simulink model "m01_PMSM_Desktop"  (R2023b)
settings: Solver=FixedStepAuto  StartTime=0.0  StopTime=0.6  FixedStep=Ts  RelTol=1e-3  AbsTol=1e-3
PreLoadFcn:
  | control_data;
  | pmsm_data;
undefined symbols (not defined in the file): avgFactor, Gs, J, Tmax, Ts, Tsc
libraries: fl_lib x54, nesl_utility x53, ee_lib x13, SimscapeFPGAHIL_lib x12, eePmsmFieldOrientedControl x1
(part 1 of 2)
Description:
  | Three-Phase PMSM Drive
settings Model: Creator=The MathWorks, Inc.  LastModifiedBy=promero
settings SolverCC: AutoScaleAbsTol=off  MaxConsecutiveMinStep=2  ZeroCrossAlgorithm=Adaptive  AlgebraicLoopSolver=TrustRegion  MaxZcPerStep=1
settings DataIOCC: MaxDataPoints=690000  SaveOutput=off  DSMLogging=off  SaveTime=off
settings OptimizationCC: ReuseModelBlockBuffer=off  LifeSpan=inf
settings DebuggingCC: UnderspecifiedInitializationDetection=Classic  MergeDetectMultiDrivingBlocksExec=none  MaxConsecutiveZCsMsg=none  IgnoredZcDiagnostic=none  InheritedTsInSrcMsg=none  UnconnectedInputMsg=warning  UnconnectedOutputMsg=warning  UnconnectedLineMsg=warning  AllowSymbolicDim=off  PregeneratedLibrarySubsystemCodeDiagnostic=none  SFUnexpectedBacktrackingDiag=warning  SFNoUnconditionalDefaultTransitionDiag=warning  SFExecutionAtInitializationDiag=none  ArithmeticOperatorsInVariantConditions=warning
settings HardwareCC: ProdBitPerPointer=32  ProdBitPerSizeT=32  ProdBitPerPtrDiffT=32  ProdLargestAtomicFloat=None  ProdIntDivRoundTo=Undefined  ProdEndianess=Unspecified  ProdWordSize=32  ProdHWDeviceType=ASIC/FPGA->ASIC/FPGA  TargetBitPerPointer=64  TargetBitPerSizeT=64  TargetBitPerPtrDiffT=64  TargetLongLongMode=on  TargetIntDivRoundTo=Zero  TargetEndianess=LittleEndian  TargetWordSize=64  TargetHWDeviceType=Custom Processor->MATLAB Host Computer  ProdEqTarget=off
settings ModelReferenceCC: EnableRefExpFcnMdlSchedulingChecks=on  PropagateSignalLabelsOutOfModel=off
settings SFSimCC: SimUseLocalCustomCode=off
settings RTWCC: RTWUseLocalCustomCode=off  DLArmComputeVersion=19.05
settings CodeAppCC: StateflowObjectComments=on
settings GRTTargetCC: TargetLangStandard=C89/C90 (ANSI)
settings ConfigComp: CovMetricSettings=dw  CovSaveCumulativeToWorkspaceVar=on  CovSaveSingleToWorkspaceVar=on  CovExternalEMLEnable=off  CovSFcnEnable=off
settings SimscapeCC: SimscapeLogSimulationStatistics=on  SimscapeLogName=simlog_ee_pmsm_drive  SimscapeLogDataHistory=690000

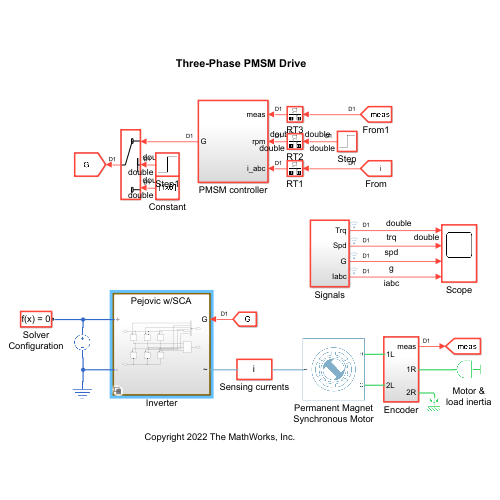
[thumbnail: Simulink's stored preview of the top-level diagram]
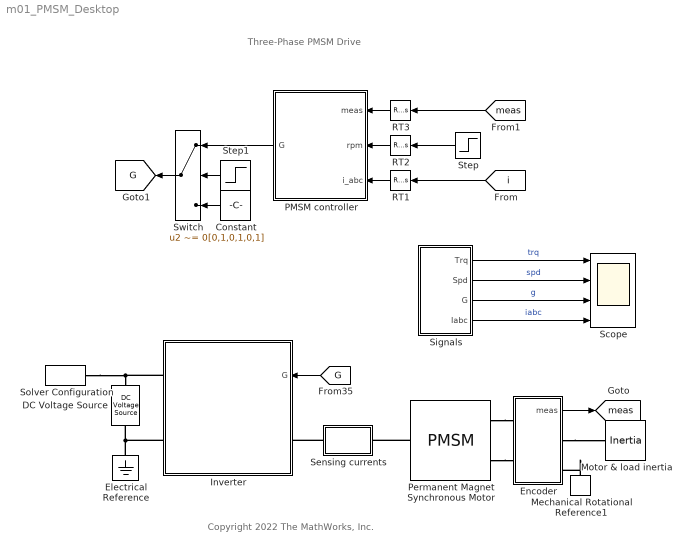
== system m01_PMSM_Desktop ==
  note: Three-Phase PMSM Drive
  note: Copyright 2022 The MathWorks, Inc.
  Constant : Constant  Value=[0,1,0,1,0,1]  SampleTime=-1
  DC Voltage Source : fl_lib/Electrical/Electrical Sources/DC Voltage Source  v0=48 V
  Electrical Reference : fl_lib/Electrical/Electrical Elements/Electrical Reference
  Encoder : Subsystem
  Inverter : Subsystem  Variant=on  VariantControlMode=label  VariantControl=Choice  LabelModeActiveChoice=PejovicSCA
  Mechanical Rotational Reference1 : fl_lib/Mechanical/Rotational Elements/Mechanical Rotational Reference
  Motor & load inertia : fl_lib/Mechanical/Rotational Elements/Inertia  inertia=J kg*m^2  num_ports=foundation.enum.numPorts2.one  w_specify=on  w_priority=High  w=0 rpm  w_nominal_specify=off  w_nominal_unit=rad/s  w_nominal_value=1  t_specify=off  t_priority=High  t=0 N*m  t_nominal_specify=off  t_nominal_unit=N*m  t_nominal_value=1
  PMSM controller : Subsystem
  Permanent Magnet Synchronous Motor : ee_lib/Electromechanical/Permanent Magnet/PMSM  port_option=ee.enum.threePhasePort.composite  winding_type=ee.enum.statorconnection.wye  machine_param=ee.enum.pmsm.parameterization.constant  nPolePairs=N  pmflux_param=ee.enum.pmflux.fluxlinkage  pm_flux_linkage=PM Wb  torque_constant=0.18 N*m/A  back_emf_constant=0.18 V/(rad/s)  stator_param=ee.enum.statorparam.LdLqL0  Ld=Ld H  Lq=Lq H  idVec=[-200, 0, 200] A  iqVec=[-200, 0, 200] A  LdMatrix=0.0002 * ones(3, 3) H  LqMatrix=0.0002 * ones(3, 3) H  PmMatrix=0.1 * ones(3, 3) Wb  ktMatrix=0.18 * ones(3, 3) N*m/A  keMatrix=0.18 * ones(3, 3) V/(rad/s)  L0=L0 H  Ls=0.0002 H  Lm=0.00002 H  Ms=0.00002 H  Rs=Rs Ohm  zero_sequence=ee.enum.park.zerosequence.exclude  axes_param=ee.enum.rotorangle.qaxis  loss_param=ee.enum.ironloss.none  losses_oc=[0, 0, 0] W  losses_sc=[0, 0, 0] W  f_losses=60 Hz  Isc_losses=95 A  J=0 kg*m^2  lam=0 N*m/(rad/s)  i_d_specify=off  i_d_priority=None  i_d=0 A  i_d_nominal_specify=off  i_d_nominal_unit=A  i_d_nominal_value=1  i_q_specify=off  i_q_priority=None  i_q=0 A  i_q_nominal_specify=off  i_q_nominal_unit=A  i_q_nominal_value=1  torque_specify=off  torque_priority=None  torque=0 N*m  torque_nominal_specify=off  torque_nominal_unit=N*m  torque_nominal_value=1  angular_velocity_specify=on  angular_velocity_priority=None  angular_velocity=0 rpm  angular_velocity_nominal_specify=off  angular_velocity_nominal_unit=rpm  angular_velocity_nominal_value=1  angular_position_specify=on  angular_position_priority=High  angular_position=0 rad  angular_position_nominal_specify=off  angular_position_nominal_unit=deg  angular_position_nominal_value=1  alpha=3.93e-3 1/K  alpha_flux=-0.001 1/K  Tmeas=298.15 K  stator_thermal_mass=100 J/K  rotor_thermal_mass=200 J/K  Rm_percent_rotor=90  Rd_percent_rotor=30  temperatureA_specify=off  temperatureA_priority=High  temperatureA=25 degC  temperatureA_nominal_specify=off  temperatureA_nominal_unit=degC  temperatureA_nominal_value=1  temperatureB_specify=off  temperatureB_priority=High  temperatureB=25 degC  temperatureB_nominal_specify=off  temperatureB_nominal_unit=degC  temperatureB_nominal_value=1  temperatureC_specify=off  temperatureC_priority=High  temperatureC=25 degC  temperatureC_nominal_specify=off  temperatureC_nominal_unit=degC  temperatureC_nominal_value=1  temperatureR_specify=off  temperatureR_priority=High  temperatureR=25 degC  temperatureR_nominal_specify=off  temperatureR_nominal_unit=degC  temperatureR_nominal_value=1
      settings: InternalSimscapePortConfiguration="{\"Bottom\":[],\"Left\":[{\"id\":\"N\",\"label\":\"~\",\"type\":\"foundation.electrical.three_phase\"}],\"Right\":[{\"id\":\"R\",\"label\":\"R\",\"type\":\"foundation.mechanical.rotational.rotational\"},{\"id\":\"C\",\"label\":\"C\",\"type\":\"foundation.mechanical.rotational.rotational\"}],\"Top\":[]}"
  RT1 : RateTransition  OutPortSampleTime=Tsc
  RT2 : RateTransition  OutPortSampleTime=Tsc
  RT3 : RateTransition  OutPortSampleTime=Tsc
  Scope : Scope  NumInputPorts=4
  Sensing currents : Subsystem
      mask Display: disp('i')
  "Signals " : Subsystem
  Solver Configuration : nesl_utility/Solver Configuration  PhysicalDomain=network_engine_domain  SubClassName=solver  LeftPortType=input  RightPortType=generic  Tones=[]  Harmonics=[]  SimulateNoise=off  Profile=off  UseLocalSampling=off  EnableSwitchedLinearOptims=on  FrequencyDomain=off  UseCCode=off  RelTol=0.001  AbsTol=1e-06  MinStep=1e-09  ToWorkspace=off  RevertToSquareIcSolve=off  NumHomotopyIterations=100  PhasorMode=off  PhasorModeNumHarmonics=1  ConsistencySolver=NEWTON_FTOL  IndexReductionMethod=DerivativeReplacement  DoDC=off  ResidualTolerance=1e-9  ConsistencyTolSource=GLOBAL  ConsistencyAbsTol=0.001  ConsistencyRelTol=0.001  ConsistencyTolFactor=0.001  UseLocalSolver=on  LocalSolverChoice=NE_PARTITIONING_ADVANCER  ResolveIndetEquations=on  FunctionEvalNumThread=1  LocalSolverSampleTime=Ts  DoFixedCost=off  MaxNonlinIter=1  MaxModeIter=2  ComputeImpulses=off  ImpulseIterations=2  LinearAlgebra=auto  LinearAlgebraNumThread=0  EquationFormulation=NE_TIME_EF  DelaysMemoryBudget=1024  AutomaticFiltering=on  FilteringTimeConstant=0.001  PartitionStorageMethod=AS_NEEDED  PartitionMemoryBudget=1024  PartitionMethod=FAST  MultibodyUseLocalSolver=off  MultibodyLocalSolverChoice=ODE1  MultibodyLocalSolverSampleTime=0.001
  Step : Step  Time=0.1  After=500  SampleTime=Tsc
  Step1 : Step  Time=1e-4
  Switch : Switch  Criteria=u2 ~= 0  SaturateOnIntegerOverflow=off  InputSameDT=off
  tag scope: G=global, meas=global
  wires:
  Step/1 -> RT2/1
  RT3/1 -> PMSM controller/1(meas)
  RT2/1 -> PMSM controller/2(rpm)
  RT1/1 -> PMSM controller/3(i_abc)
  "Signals "/2(Spd) -> Scope/2  "spd"
  "Signals "/4(Iabc) -> Scope/4  "iabc"
  "Signals "/3(G) -> Scope/3  "g"
  "Signals "/1(Trq) -> Scope/1  "trq"
  [i] -> RT1/1
  Encoder/1(meas) -> [meas]
  [meas] -> RT3/1
  PMSM controller/1(G) -> Switch/1
  Constant/1 -> Switch/3
  Step1/1 -> Switch/2
  Switch/1 -> [G]
  [G] -> Inverter/1(G)
  connections:
  Permanent Magnet Synchronous Motor/RConn1 -- Encoder/LConn1
  Permanent Magnet Synchronous Motor/RConn2 -- Encoder/LConn2
  Encoder/RConn1 -- Motor & load inertia/LConn1
  Mechanical Rotational Reference1/LConn1 -- Encoder/RConn2
  Permanent Magnet Synchronous Motor/LConn1 -- Sensing currents/RConn1
  Solver Configuration/RConn1 -- DC Voltage Source/LConn1 -- Inverter/RConn1
  DC Voltage Source/RConn1 -- Inverter/RConn2 -- Electrical Reference/LConn1
  Sensing currents/LConn1 -- Inverter/LConn1

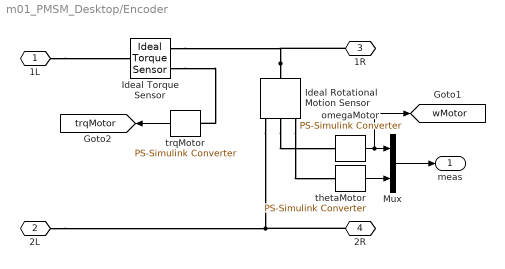
== system m01_PMSM_Desktop/Encoder ==
  Ideal Rotational Motion Sensor : fl_lib/Mechanical/Mechanical Sensors/Ideal Rotational Motion Sensor  reference=foundation.enum.MeasurementReference.difference  acceleration_port=false  velocity_port=true  position_port=true  wrap_angle=simscape.enum.onoff.off  offset=0 deg
  Ideal Torque Sensor : fl_lib/Mechanical/Mechanical Sensors/Ideal Torque Sensor
  Mux : Mux  Inputs=2
  omegaMotor : nesl_utility/PS-Simulink Converter  PhysicalDomain=network_engine_domain  SubClassName=ps_output  LeftPortType=input  RightPortType=output  PseudoPeriodic=off  Frequencies=[]  VectorFormat=1-D array  Unit=inherit  AffineConversion=off
  thetaMotor : nesl_utility/PS-Simulink Converter  PhysicalDomain=network_engine_domain  SubClassName=ps_output  LeftPortType=input  RightPortType=output  PseudoPeriodic=off  Frequencies=[]  VectorFormat=1-D array  Unit=inherit  AffineConversion=off
  trqMotor : nesl_utility/PS-Simulink Converter  PhysicalDomain=network_engine_domain  SubClassName=ps_output  LeftPortType=input  RightPortType=output  PseudoPeriodic=off  Frequencies=[]  VectorFormat=1-D array  Unit=inherit  AffineConversion=off
  1L : PMIOPort  Side=Left
  2L : PMIOPort  Port=2  Side=Left
  1R : PMIOPort  Port=3  Side=Right
  2R : PMIOPort  Port=4  Side=Right
  meas : Outport  VectorParamsAs1DForOutWhenUnconnected=off
  tag scope: trqMotor=global, wMotor=global
  wires:
  trqMotor/1 -> [trqMotor]
  Mux/1 -> meas/1
  thetaMotor/1 -> Mux/2
  omegaMotor/1 -> [wMotor], Mux/1
  connections:
  Ideal Torque Sensor/RConn2 -- trqMotor/LConn1
  1L/RConn1 -- Ideal Torque Sensor/LConn1
  2R/RConn1 -- 2L/RConn1 -- Ideal Rotational Motion Sensor/RConn1
  Ideal Rotational Motion Sensor/LConn1 -- 1R/RConn1 -- Ideal Torque Sensor/RConn1
  Ideal Rotational Motion Sensor/RConn2 -- omegaMotor/LConn1
  Ideal Rotational Motion Sensor/RConn3 -- thetaMotor/LConn1

== system m01_PMSM_Desktop/Inverter ==
  G : Inport
  Pejovic : Subsystem  VariantControl=Pejovic
  Pejovic w/SCA : Subsystem  VariantControl=PejovicSCA
  Simscape Converter : Subsystem  VariantControl=SimscapeConv
  Simscape Switches : Subsystem  VariantControl=SimscapeSw
  + : PMIOPort  Side=Right
  - : PMIOPort  Port=2  Side=Right
  ~ : PMIOPort  Port=3  Side=Left

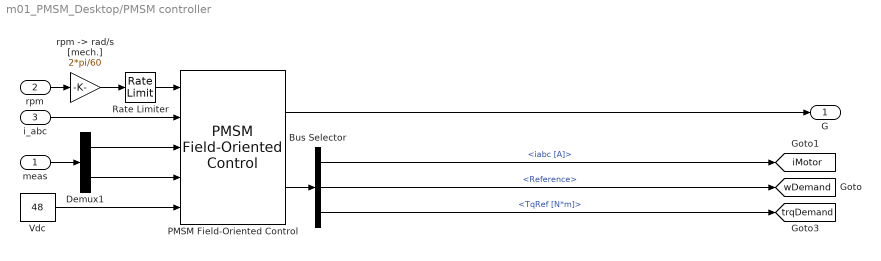
== system m01_PMSM_Desktop/PMSM controller ==
  meas : Inport
  rpm : Inport  Port=2
  i_abc : Inport  Port=3
  Bus Selector : BusSelector  OutputSignals=iabc [A],Reference,TqRef [N*m]
  Demux1 : Demux  Outputs=2
  PMSM Field-Oriented Control : eePmsmFieldOrientedControl/PMSM Field-Oriented Control  winding_type=Wye-wound  CtrlMode=Velocity control  Vnom=48  Pmax=Pmax  Tmax=Tmax*1.5  p=N  Vdc_on=10  Ts=Ts  Tsc=Tsc  CtrlType=PI control  Kp_w=60  Ki_w=300*2  Kv_w=1  Kaw_w=1000  RefType=Zero d-axis control  rpmVec=[0, 3000]  TqVec=[-100, 0, 100]  VdcVec=[300, 350]  PWMMode=SPWM: sinusoidal PWM  ModFactor=1  idMatrix=zeros(2,3,2)  iqMatrix=zeros(2,3,2)  psim=PM  Ld=0.00024  Lq=0.00029  Rs=0.01  AxisAlignment=Q-axis  Kp_id=0.1  Ki_id=10  Kaw_id=1000  Kp_iq=0.1  Ki_iq=10  Kaw_iq=1000  AxisPrio=Q-axis  ActZC=off  ActFF=on  ParamTypeFF=Constant parameters  LdFF=Ld  LqFF=Lq  psimFF=PM  idVect=[-200, 0, 200]  iqVect=[-200, 0, 200]  LdMatrix=0.0002 * ones(3, 3)  LqMatrix=0.0002 * ones(3, 3)  psimMatrix=0.04 * ones(3, 3)  CPWMMode=SPWM: sinusoidal PWM  fsw=fsw
  Rate Limiter : RateLimiter  RisingSlewLimit=Tmax/J  FallingSlewLimit=-Tmax/J  SampleTimeMode=inherited
  Vdc : Constant  Value=48  SampleTime=Tsc
  "rpm -> rad/s [mech.]" : Gain  Gain=2*pi/60
  G : Outport  VectorParamsAs1DForOutWhenUnconnected=off
  tag scope: iMotor=global, trqDemand=global, wDemand=global
  wires:
  Vdc/1 -> PMSM Field-Oriented Control/5
  PMSM Field-Oriented Control/2 -> Bus Selector/1
  i_abc/1 -> PMSM Field-Oriented Control/2
  meas/1 -> Demux1/1
  Demux1/1 -> PMSM Field-Oriented Control/3
  Demux1/2 -> PMSM Field-Oriented Control/4
  Bus Selector/1 -> [iMotor]  "<iabc [A]>"
  Bus Selector/2 -> [wDemand]  "<Reference>"
  Bus Selector/3 -> [trqDemand]  "<TqRef [N*m]>"
  rpm/1 -> "rpm -> rad/s [mech.]"/1
  Rate Limiter/1 -> PMSM Field-Oriented Control/1
  "rpm -> rad/s [mech.]"/1 -> Rate Limiter/1
  PMSM Field-Oriented Control/1 -> G/1

== system m01_PMSM_Desktop/Sensing currents ==
  Current Sensor : ee_lib/Sensors & Transducers/Current Sensor (Three-Phase)
  Gain : Gain  Commented=through  Gain=1/sqrt(3)
  Iabc : nesl_utility/PS-Simulink Converter  PhysicalDomain=network_engine_domain  SubClassName=ps_output  LeftPortType=input  RightPortType=output  PseudoPeriodic=off  Frequencies=[]  VectorFormat=1-D array  Unit=A  AffineConversion=off
  Conn1 : PMIOPort  Side=Left
  Conn2 : PMIOPort  Port=2  Side=Right
  tag scope: i=global
  wires:
  Iabc/1 -> Gain/1
  Gain/1 -> [i]
  connections:
  Current Sensor/RConn1 -- Iabc/LConn1
  Conn2/RConn1 -- Current Sensor/RConn2
  Current Sensor/LConn1 -- Conn1/RConn1

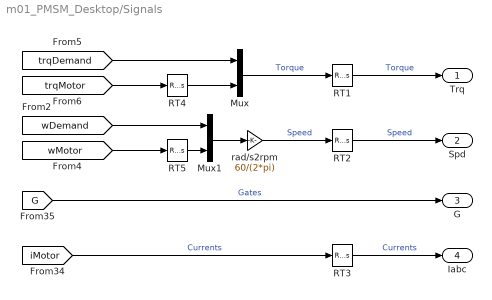
== system m01_PMSM_Desktop/Signals  ==
  Mux : Mux  Inputs=2
  Mux1 : Mux  Inputs=2
  RT1 : RateTransition  OutPortSampleTime=Ts
  RT2 : RateTransition  OutPortSampleTime=Ts
  RT3 : RateTransition  OutPortSampleTime=Ts
  RT4 : RateTransition  OutPortSampleTime=Tsc
  RT5 : RateTransition  OutPortSampleTime=Tsc
  rad/s2rpm : Gain  Gain=60/(2*pi)
  Trq : Outport  VectorParamsAs1DForOutWhenUnconnected=off
  Spd : Outport  Port=2  VectorParamsAs1DForOutWhenUnconnected=off
  G : Outport  Port=3  VectorParamsAs1DForOutWhenUnconnected=off
  Iabc : Outport  Port=4  VectorParamsAs1DForOutWhenUnconnected=off
  wires:
  [trqDemand] -> Mux/1
  [G] -> G/1  "Gates"
  Mux1/1 -> rad/s2rpm/1
  Mux/1 -> RT1/1  "Torque"
  [iMotor] -> RT3/1  "Currents"
  [wDemand] -> Mux1/1
  rad/s2rpm/1 -> RT2/1  "Speed"
  [trqMotor] -> RT4/1
  [wMotor] -> RT5/1
  RT1/1 -> Trq/1  "Torque"
  RT2/1 -> Spd/1  "Speed"
  RT3/1 -> Iabc/1  "Currents"
  RT4/1 -> Mux/2
  RT5/1 -> Mux1/2

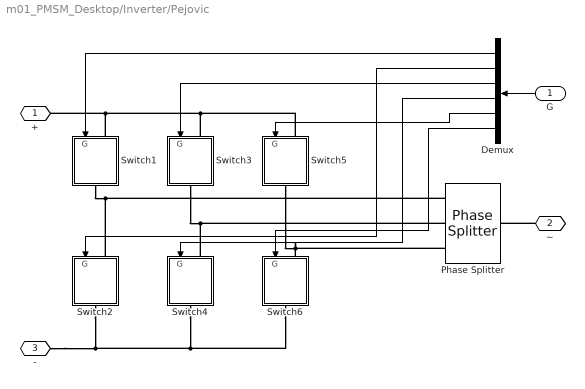
== system m01_PMSM_Desktop/Inverter/Pejovic ==
  G : Inport
  Demux : Demux  Outputs=6
  Phase Splitter : ee_lib/Connectors & References/Phase Splitter
  Switch1 : Subsystem  mask{threshold=0.5, Gs=Gs, timeScaling=1, avgFactor=1}
      mask prompts: threshold "Threshold voltage [V]"; Gs "Conductance (1/Ohm)"; timeScaling "Time scaling"; avgFactor "Subcycle average factor"
      settings: CopyFcn=set_param(gcb, 'LinkStatus', 'none');
  Switch2 : Subsystem  mask{threshold=0.5, Gs=Gs, timeScaling=1, avgFactor=1}
      mask prompts: threshold "Threshold voltage [V]"; Gs "Conductance (1/Ohm)"; timeScaling "Time scaling"; avgFactor "Subcycle average factor"
      settings: CopyFcn=set_param(gcb, 'LinkStatus', 'none');
  Switch3 : Subsystem  mask{threshold=0.5, Gs=Gs, timeScaling=1, avgFactor=1}
      mask prompts: threshold "Threshold voltage [V]"; Gs "Conductance (1/Ohm)"; timeScaling "Time scaling"; avgFactor "Subcycle average factor"
      settings: CopyFcn=set_param(gcb, 'LinkStatus', 'none');
  Switch4 : Subsystem  mask{threshold=0.5, Gs=Gs, timeScaling=1, avgFactor=1}
      mask prompts: threshold "Threshold voltage [V]"; Gs "Conductance (1/Ohm)"; timeScaling "Time scaling"; avgFactor "Subcycle average factor"
      settings: CopyFcn=set_param(gcb, 'LinkStatus', 'none');
  Switch5 : Subsystem  mask{threshold=0.5, Gs=Gs, timeScaling=1, avgFactor=1}
      mask prompts: threshold "Threshold voltage [V]"; Gs "Conductance (1/Ohm)"; timeScaling "Time scaling"; avgFactor "Subcycle average factor"
      settings: CopyFcn=set_param(gcb, 'LinkStatus', 'none');
  Switch6 : Subsystem  mask{threshold=0.5, Gs=Gs, timeScaling=1, avgFactor=1}
      mask prompts: threshold "Threshold voltage [V]"; Gs "Conductance (1/Ohm)"; timeScaling "Time scaling"; avgFactor "Subcycle average factor"
      settings: CopyFcn=set_param(gcb, 'LinkStatus', 'none');
  + : PMIOPort  Side=Right
  ~ : PMIOPort  Port=2  Side=Left
  - : PMIOPort  Port=3  Side=Right
  wires:
  Demux/6 -> Switch6/1(G)
  Demux/5 -> Switch5/1(G)
  Demux/4 -> Switch4/1(G)
  Demux/3 -> Switch3/1(G)
  Demux/2 -> Switch2/1(G)
  Demux/1 -> Switch1/1(G)
  G/1 -> Demux/1
  connections:
  +/RConn1 -- Switch1/LConn1 -- Switch5/LConn1 -- Switch3/LConn1
  Phase Splitter/RConn1 -- Switch2/LConn1 -- Switch1/RConn1
  Switch6/RConn1 -- Switch4/RConn1 -- Switch2/RConn1 -- -/RConn1
  ~/RConn1 -- Phase Splitter/LConn1
  Phase Splitter/RConn2 -- Switch4/LConn1 -- Switch3/RConn1
  Phase Splitter/RConn3 -- Switch6/LConn1 -- Switch5/RConn1

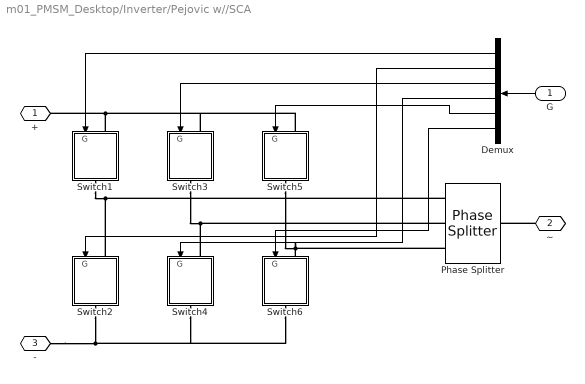
== system m01_PMSM_Desktop/Inverter/Pejovic w//SCA ==
  G : Inport
  Demux : Demux  Outputs=6
  Phase Splitter : ee_lib/Connectors & References/Phase Splitter
  Switch1 : Subsystem  mask{threshold=0.5, Gs=Gs, timeScaling=1, avgFactor=avgFactor}
      mask prompts: threshold "Threshold voltage [V]"; Gs "Conductance (1/Ohm)"; timeScaling "Time scaling"; avgFactor "Subcycle average factor"
      settings: CopyFcn=set_param(gcb, 'LinkStatus', 'none');
  Switch2 : Subsystem  mask{threshold=0.5, Gs=Gs, timeScaling=1, avgFactor=avgFactor}
      mask prompts: threshold "Threshold voltage [V]"; Gs "Conductance (1/Ohm)"; timeScaling "Time scaling"; avgFactor "Subcycle average factor"
      settings: CopyFcn=set_param(gcb, 'LinkStatus', 'none');
  Switch3 : Subsystem  mask{threshold=0.5, Gs=Gs, timeScaling=1, avgFactor=avgFactor}
      mask prompts: threshold "Threshold voltage [V]"; Gs "Conductance (1/Ohm)"; timeScaling "Time scaling"; avgFactor "Subcycle average factor"
      settings: CopyFcn=set_param(gcb, 'LinkStatus', 'none');
  Switch4 : Subsystem  mask{threshold=0.5, Gs=Gs, timeScaling=1, avgFactor=avgFactor}
      mask prompts: threshold "Threshold voltage [V]"; Gs "Conductance (1/Ohm)"; timeScaling "Time scaling"; avgFactor "Subcycle average factor"
      settings: CopyFcn=set_param(gcb, 'LinkStatus', 'none');
  Switch5 : Subsystem  mask{threshold=0.5, Gs=Gs, timeScaling=1, avgFactor=avgFactor}
      mask prompts: threshold "Threshold voltage [V]"; Gs "Conductance (1/Ohm)"; timeScaling "Time scaling"; avgFactor "Subcycle average factor"
      settings: CopyFcn=set_param(gcb, 'LinkStatus', 'none');
  Switch6 : Subsystem  mask{threshold=0.5, Gs=Gs, timeScaling=1, avgFactor=avgFactor}
      mask prompts: threshold "Threshold voltage [V]"; Gs "Conductance (1/Ohm)"; timeScaling "Time scaling"; avgFactor "Subcycle average factor"
      settings: CopyFcn=set_param(gcb, 'LinkStatus', 'none');
  + : PMIOPort  Side=Right
  ~ : PMIOPort  Port=2  Side=Left
  - : PMIOPort  Port=3  Side=Right
  wires:
  G/1 -> Demux/1
  Demux/1 -> Switch1/1(G)
  Demux/2 -> Switch2/1(G)
  Demux/3 -> Switch3/1(G)
  Demux/4 -> Switch4/1(G)
  Demux/5 -> Switch5/1(G)
  Demux/6 -> Switch6/1(G)
  connections:
  Phase Splitter/RConn3 -- Switch6/LConn1 -- Switch5/RConn1
  Phase Splitter/RConn2 -- Switch4/LConn1 -- Switch3/RConn1
  ~/RConn1 -- Phase Splitter/LConn1
  Switch6/RConn1 -- Switch4/RConn1 -- Switch2/RConn1 -- -/RConn1
  Phase Splitter/RConn1 -- Switch2/LConn1 -- Switch1/RConn1
  Switch5/LConn1 -- Switch3/LConn1 -- Switch1/LConn1 -- +/RConn1

== system m01_PMSM_Desktop/Inverter/Simscape Converter ==
  G : Inport
  Converter (Three-Phase) : ee_lib/Semiconductors & Converters/Converters/Converter (Three-Phase)  port_option=ee.enum.threePhasePort.composite  device_type=ee.enum.converters.switchingdevice.ideal  K=0  Vf=0.8 V  Ron=0.001 Ohm  Rds=0.001 Ohm  Goff=1e-6 1/Ohm  Vgt=1 V  Vgt_off=-1 V  Ih=1 A  Vth=0.5 V  diode_param=ee.enum.converters.protectiondiode.none  diode_Vf=0.8 V  diode_Ron=0.001 Ohm  diode_Goff=1e-5 1/Ohm  diode_C=50 nF  diode_iRM=-235 A  diode_iF=300 A  diode_idot=-50 A/us  diode_trr_param=ee.enum.converters.diodetrr.trr_factor  diode_trr_factor=3  diode_trr=15 us  diode_Qrr=1500 s*uA  snubber_type=ee.enum.converters.snubber.exclude  Cs=1e-7 F  Rs=0.1 Ohm
  Gates : Subsystem
  + : PMIOPort  Side=Right
  ~ : PMIOPort  Port=2  Side=Left
  - : PMIOPort  Port=3  Side=Right
  wires:
  G/1 -> Gates/1(Gates Simulink)
  connections:
  -/RConn1 -- Converter (Three-Phase)/RConn2
  Converter (Three-Phase)/RConn1 -- +/RConn1
  Gates/RConn1 -- Converter (Three-Phase)/LConn1
  Converter (Three-Phase)/LConn2 -- ~/RConn1

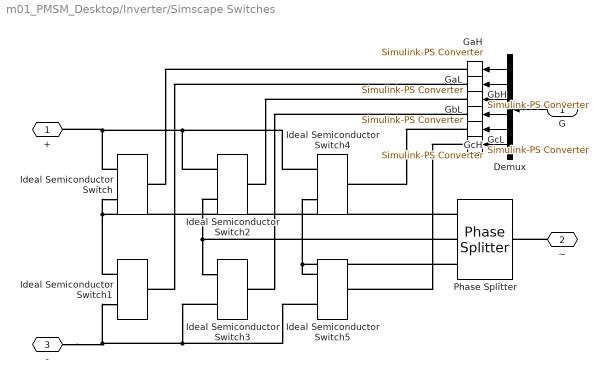
== system m01_PMSM_Desktop/Inverter/Simscape Switches ==
  G : Inport
  Demux : Demux  Outputs=6
  GaH : nesl_utility/Simulink-PS Converter  PhysicalDomain=network_engine_domain  SubClassName=ps_input  LeftPortType=input  RightPortType=output  PseudoPeriodic=off  Frequencies=[]  NoiseDistribution=none  NoiseParameters=[]  Unit=1  AffineConversion=off  FilteringAndDerivatives=zero  SimscapeFilterOrder=1  InputFilterTimeConstant=0.001  UdotUserProvided=0
  GaL : nesl_utility/Simulink-PS Converter  PhysicalDomain=network_engine_domain  SubClassName=ps_input  LeftPortType=input  RightPortType=output  PseudoPeriodic=off  Frequencies=[]  NoiseDistribution=none  NoiseParameters=[]  Unit=1  AffineConversion=off  FilteringAndDerivatives=zero  SimscapeFilterOrder=1  InputFilterTimeConstant=0.001  UdotUserProvided=0
  GbH : nesl_utility/Simulink-PS Converter  PhysicalDomain=network_engine_domain  SubClassName=ps_input  LeftPortType=input  RightPortType=output  PseudoPeriodic=off  Frequencies=[]  NoiseDistribution=none  NoiseParameters=[]  Unit=1  AffineConversion=off  FilteringAndDerivatives=zero  SimscapeFilterOrder=1  InputFilterTimeConstant=0.001  UdotUserProvided=0
  GbL : nesl_utility/Simulink-PS Converter  PhysicalDomain=network_engine_domain  SubClassName=ps_input  LeftPortType=input  RightPortType=output  PseudoPeriodic=off  Frequencies=[]  NoiseDistribution=none  NoiseParameters=[]  Unit=1  AffineConversion=off  FilteringAndDerivatives=zero  SimscapeFilterOrder=1  InputFilterTimeConstant=0.001  UdotUserProvided=0
  GcH : nesl_utility/Simulink-PS Converter  PhysicalDomain=network_engine_domain  SubClassName=ps_input  LeftPortType=input  RightPortType=output  PseudoPeriodic=off  Frequencies=[]  NoiseDistribution=none  NoiseParameters=[]  Unit=1  AffineConversion=off  FilteringAndDerivatives=zero  SimscapeFilterOrder=1  InputFilterTimeConstant=0.001  UdotUserProvided=0
  GcL : nesl_utility/Simulink-PS Converter  PhysicalDomain=network_engine_domain  SubClassName=ps_input  LeftPortType=input  RightPortType=output  PseudoPeriodic=off  Frequencies=[]  NoiseDistribution=none  NoiseParameters=[]  Unit=1  AffineConversion=off  FilteringAndDerivatives=zero  SimscapeFilterOrder=1  InputFilterTimeConstant=0.001  UdotUserProvided=0
  Ideal Semiconductor Switch{,1..5} (6 alike) : ee_lib/Semiconductors & Converters/Ideal Semiconductor Switch  port_option=ee.enum.controlport.ps  Ron=0.001 Ohm  Goff=1e-6 1/Ohm  Vth=0.5 V  diode_param=ee.enum.converters.protectiondiode.none  diode_Vf=0.8 V  diode_Ron=0.001 Ohm  diode_Goff=1e-5 1/Ohm  diode_C=50e-9 F  diode_iRM=-235 A  diode_iF=300 A  diode_idot=-50 A/us  diode_trr_param=ee.enum.converters.diodetrr.trr_factor  diode_trr_factor=3  diode_trr=15 us  diode_Qrr=1500 s*uA
  Phase Splitter : ee_lib/Connectors & References/Phase Splitter
  + : PMIOPort  Side=Right
  ~ : PMIOPort  Port=2  Side=Left
  - : PMIOPort  Port=3  Side=Right
  wires:
  Demux/6 -> GcL/1
  Demux/2 -> GaL/1
  Demux/3 -> GbH/1
  Demux/5 -> GcH/1
  Demux/4 -> GbL/1
  Demux/1 -> GaH/1
  G/1 -> Demux/1
  connections:
  Ideal Semiconductor Switch/RConn1 -- Ideal Semiconductor Switch4/RConn1 -- Ideal Semiconductor Switch2/RConn1 -- +/RConn1
  Ideal Semiconductor Switch1/RConn1 -- Phase Splitter/RConn1 -- Ideal Semiconductor Switch/RConn2
  -/RConn1 -- Ideal Semiconductor Switch5/RConn2 -- Ideal Semiconductor Switch3/RConn2 -- Ideal Semiconductor Switch1/RConn2
  ~/RConn1 -- Phase Splitter/LConn1
  Ideal Semiconductor Switch2/RConn2 -- Ideal Semiconductor Switch3/RConn1 -- Phase Splitter/RConn2
  Ideal Semiconductor Switch5/RConn1 -- Ideal Semiconductor Switch4/RConn2 -- Phase Splitter/RConn3
  GaH/RConn1 -- Ideal Semiconductor Switch/LConn1
  GaL/RConn1 -- Ideal Semiconductor Switch1/LConn1
  GbH/RConn1 -- Ideal Semiconductor Switch2/LConn1
  GbL/RConn1 -- Ideal Semiconductor Switch3/LConn1
  GcH/RConn1 -- Ideal Semiconductor Switch4/LConn1
  GcL/RConn1 -- Ideal Semiconductor Switch5/LConn1

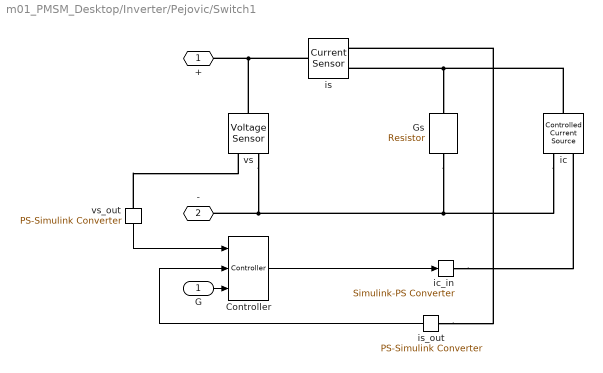
== system m01_PMSM_Desktop/Inverter/Pejovic/Switch1 ==
  G : Inport
  Controller : SimscapeFPGAHIL_lib/Linearized Switch Models/Switch/Controller  threshold=threshold  Gs=Gs  s=timeScaling  avgFactor=avgFactor  isFixedPoint=off
  Gs : fl_lib/Electrical/Electrical Elements/Resistor  R=1/Gs Ohm  i_specify=off  i_priority=None  i=0 A  i_nominal_specify=off  i_nominal_unit=A  i_nominal_value=1  v_specify=off  v_priority=None  v=0 V  v_nominal_specify=off  v_nominal_unit=V  v_nominal_value=1
      settings: LibrarySourceBlock=SimscapeFPGAHIL_lib/Linearized Switch Models/Switch/Gs
  ic : fl_lib/Electrical/Electrical Sources/Controlled Current Source
      settings: LibrarySourceBlock=SimscapeFPGAHIL_lib/Linearized Switch Models/Switch/ic
  ic_in : nesl_utility/Simulink-PS Converter  PhysicalDomain=network_engine_domain  SubClassName=ps_input  LeftPortType=input  RightPortType=output  PseudoPeriodic=off  Frequencies=[]  NoiseDistribution=none  NoiseParameters=[]  Unit=A  AffineConversion=off  FilteringAndDerivatives=provide  SimscapeFilterOrder=1  InputFilterTimeConstant=0.001  UdotUserProvided=0
      settings: LibrarySourceBlock=SimscapeFPGAHIL_lib/Linearized Switch Models/Switch/ic_in
  is : fl_lib/Electrical/Electrical Sensors/Current Sensor
      settings: LibrarySourceBlock=SimscapeFPGAHIL_lib/Linearized Switch Models/Switch/is
  is_out : nesl_utility/PS-Simulink Converter  PhysicalDomain=network_engine_domain  SubClassName=ps_output  LeftPortType=input  RightPortType=output  PseudoPeriodic=off  Frequencies=[]  VectorFormat=1-D array  Unit=A  AffineConversion=off
      settings: LibrarySourceBlock=SimscapeFPGAHIL_lib/Linearized Switch Models/Switch/is_out
  vs : fl_lib/Electrical/Electrical Sensors/Voltage Sensor
      settings: LibrarySourceBlock=SimscapeFPGAHIL_lib/Linearized Switch Models/Switch/vs
  vs_out : nesl_utility/PS-Simulink Converter  PhysicalDomain=network_engine_domain  SubClassName=ps_output  LeftPortType=input  RightPortType=output  PseudoPeriodic=off  Frequencies=[]  VectorFormat=1-D array  Unit=V  AffineConversion=off
      settings: LibrarySourceBlock=SimscapeFPGAHIL_lib/Linearized Switch Models/Switch/vs_out
  + : PMIOPort  Side=Left
  - : PMIOPort  Port=2  Side=Right
  wires:
  vs_out/1 -> Controller/1
  is_out/1 -> Controller/2
  G/1 -> Controller/3
  Controller/1 -> ic_in/1
  connections:
  ic/LConn1 -- Gs/LConn1 -- is/RConn2
  vs/RConn2 -- -/RConn1 -- Gs/RConn1 -- ic/RConn2
  vs/LConn1 -- +/RConn1 -- is/LConn1
  ic_in/RConn1 -- ic/RConn1
  vs_out/LConn1 -- vs/RConn1
  is_out/LConn1 -- is/RConn1

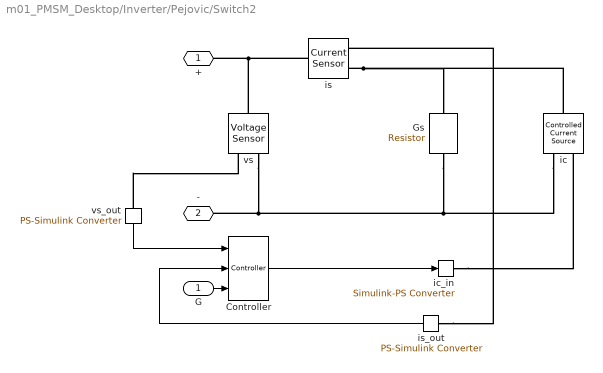
== system m01_PMSM_Desktop/Inverter/Pejovic/Switch2 ==
  G : Inport
  Controller : SimscapeFPGAHIL_lib/Linearized Switch Models/Switch/Controller  threshold=threshold  Gs=Gs  s=timeScaling  avgFactor=avgFactor  isFixedPoint=off
  Gs : fl_lib/Electrical/Electrical Elements/Resistor  R=1/Gs Ohm  i_specify=off  i_priority=None  i=0 A  i_nominal_specify=off  i_nominal_unit=A  i_nominal_value=1  v_specify=off  v_priority=None  v=0 V  v_nominal_specify=off  v_nominal_unit=V  v_nominal_value=1
      settings: LibrarySourceBlock=SimscapeFPGAHIL_lib/Linearized Switch Models/Switch/Gs
  ic : fl_lib/Electrical/Electrical Sources/Controlled Current Source
      settings: LibrarySourceBlock=SimscapeFPGAHIL_lib/Linearized Switch Models/Switch/ic
  ic_in : nesl_utility/Simulink-PS Converter  PhysicalDomain=network_engine_domain  SubClassName=ps_input  LeftPortType=input  RightPortType=output  PseudoPeriodic=off  Frequencies=[]  NoiseDistribution=none  NoiseParameters=[]  Unit=A  AffineConversion=off  FilteringAndDerivatives=provide  SimscapeFilterOrder=1  InputFilterTimeConstant=0.001  UdotUserProvided=0
      settings: LibrarySourceBlock=SimscapeFPGAHIL_lib/Linearized Switch Models/Switch/ic_in
  is : fl_lib/Electrical/Electrical Sensors/Current Sensor
      settings: LibrarySourceBlock=SimscapeFPGAHIL_lib/Linearized Switch Models/Switch/is
  is_out : nesl_utility/PS-Simulink Converter  PhysicalDomain=network_engine_domain  SubClassName=ps_output  LeftPortType=input  RightPortType=output  PseudoPeriodic=off  Frequencies=[]  VectorFormat=1-D array  Unit=A  AffineConversion=off
      settings: LibrarySourceBlock=SimscapeFPGAHIL_lib/Linearized Switch Models/Switch/is_out
  vs : fl_lib/Electrical/Electrical Sensors/Voltage Sensor
      settings: LibrarySourceBlock=SimscapeFPGAHIL_lib/Linearized Switch Models/Switch/vs
  vs_out : nesl_utility/PS-Simulink Converter  PhysicalDomain=network_engine_domain  SubClassName=ps_output  LeftPortType=input  RightPortType=output  PseudoPeriodic=off  Frequencies=[]  VectorFormat=1-D array  Unit=V  AffineConversion=off
      settings: LibrarySourceBlock=SimscapeFPGAHIL_lib/Linearized Switch Models/Switch/vs_out
  + : PMIOPort  Side=Left
  - : PMIOPort  Port=2  Side=Right
  wires:
  Controller/1 -> ic_in/1
  G/1 -> Controller/3
  is_out/1 -> Controller/2
  vs_out/1 -> Controller/1
  connections:
  is_out/LConn1 -- is/RConn1
  vs_out/LConn1 -- vs/RConn1
  ic_in/RConn1 -- ic/RConn1
  is/LConn1 -- +/RConn1 -- vs/LConn1
  ic/RConn2 -- Gs/RConn1 -- -/RConn1 -- vs/RConn2
  is/RConn2 -- Gs/LConn1 -- ic/LConn1

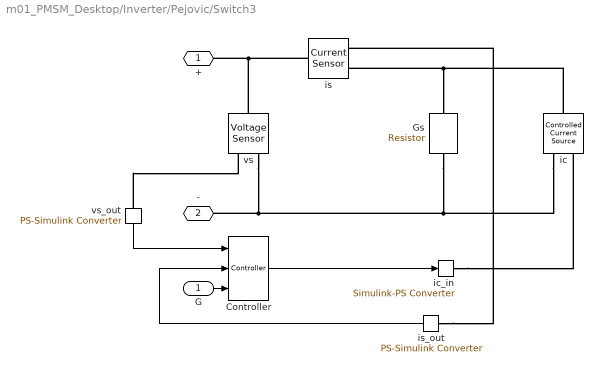
== system m01_PMSM_Desktop/Inverter/Pejovic/Switch3 ==
  G : Inport
  Controller : SimscapeFPGAHIL_lib/Linearized Switch Models/Switch/Controller  threshold=threshold  Gs=Gs  s=timeScaling  avgFactor=avgFactor  isFixedPoint=off
  Gs : fl_lib/Electrical/Electrical Elements/Resistor  R=1/Gs Ohm  i_specify=off  i_priority=None  i=0 A  i_nominal_specify=off  i_nominal_unit=A  i_nominal_value=1  v_specify=off  v_priority=None  v=0 V  v_nominal_specify=off  v_nominal_unit=V  v_nominal_value=1
      settings: LibrarySourceBlock=SimscapeFPGAHIL_lib/Linearized Switch Models/Switch/Gs
  ic : fl_lib/Electrical/Electrical Sources/Controlled Current Source
      settings: LibrarySourceBlock=SimscapeFPGAHIL_lib/Linearized Switch Models/Switch/ic
  ic_in : nesl_utility/Simulink-PS Converter  PhysicalDomain=network_engine_domain  SubClassName=ps_input  LeftPortType=input  RightPortType=output  PseudoPeriodic=off  Frequencies=[]  NoiseDistribution=none  NoiseParameters=[]  Unit=A  AffineConversion=off  FilteringAndDerivatives=provide  SimscapeFilterOrder=1  InputFilterTimeConstant=0.001  UdotUserProvided=0
      settings: LibrarySourceBlock=SimscapeFPGAHIL_lib/Linearized Switch Models/Switch/ic_in
  is : fl_lib/Electrical/Electrical Sensors/Current Sensor
      settings: LibrarySourceBlock=SimscapeFPGAHIL_lib/Linearized Switch Models/Switch/is
  is_out : nesl_utility/PS-Simulink Converter  PhysicalDomain=network_engine_domain  SubClassName=ps_output  LeftPortType=input  RightPortType=output  PseudoPeriodic=off  Frequencies=[]  VectorFormat=1-D array  Unit=A  AffineConversion=off
      settings: LibrarySourceBlock=SimscapeFPGAHIL_lib/Linearized Switch Models/Switch/is_out
  vs : fl_lib/Electrical/Electrical Sensors/Voltage Sensor
      settings: LibrarySourceBlock=SimscapeFPGAHIL_lib/Linearized Switch Models/Switch/vs
  vs_out : nesl_utility/PS-Simulink Converter  PhysicalDomain=network_engine_domain  SubClassName=ps_output  LeftPortType=input  RightPortType=output  PseudoPeriodic=off  Frequencies=[]  VectorFormat=1-D array  Unit=V  AffineConversion=off
      settings: LibrarySourceBlock=SimscapeFPGAHIL_lib/Linearized Switch Models/Switch/vs_out
  + : PMIOPort  Side=Left
  - : PMIOPort  Port=2  Side=Right
  wires:
  vs_out/1 -> Controller/1
  is_out/1 -> Controller/2
  G/1 -> Controller/3
  Controller/1 -> ic_in/1
  connections:
  ic/LConn1 -- Gs/LConn1 -- is/RConn2
  vs/RConn2 -- -/RConn1 -- Gs/RConn1 -- ic/RConn2
  vs/LConn1 -- +/RConn1 -- is/LConn1
  ic_in/RConn1 -- ic/RConn1
  vs_out/LConn1 -- vs/RConn1
  is_out/LConn1 -- is/RConn1

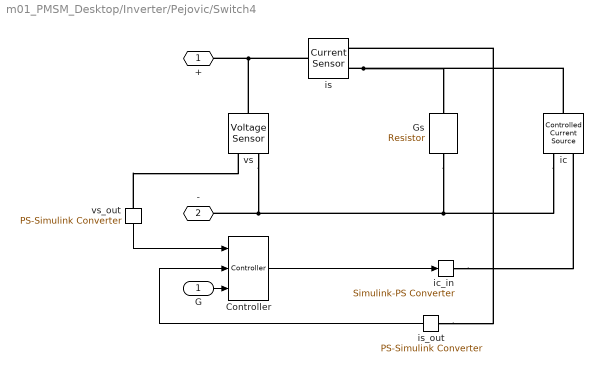
== system m01_PMSM_Desktop/Inverter/Pejovic/Switch4 ==
  G : Inport
  Controller : SimscapeFPGAHIL_lib/Linearized Switch Models/Switch/Controller  threshold=threshold  Gs=Gs  s=timeScaling  avgFactor=avgFactor  isFixedPoint=off
  Gs : fl_lib/Electrical/Electrical Elements/Resistor  R=1/Gs Ohm  i_specify=off  i_priority=None  i=0 A  i_nominal_specify=off  i_nominal_unit=A  i_nominal_value=1  v_specify=off  v_priority=None  v=0 V  v_nominal_specify=off  v_nominal_unit=V  v_nominal_value=1
      settings: LibrarySourceBlock=SimscapeFPGAHIL_lib/Linearized Switch Models/Switch/Gs
  ic : fl_lib/Electrical/Electrical Sources/Controlled Current Source
      settings: LibrarySourceBlock=SimscapeFPGAHIL_lib/Linearized Switch Models/Switch/ic
  ic_in : nesl_utility/Simulink-PS Converter  PhysicalDomain=network_engine_domain  SubClassName=ps_input  LeftPortType=input  RightPortType=output  PseudoPeriodic=off  Frequencies=[]  NoiseDistribution=none  NoiseParameters=[]  Unit=A  AffineConversion=off  FilteringAndDerivatives=provide  SimscapeFilterOrder=1  InputFilterTimeConstant=0.001  UdotUserProvided=0
      settings: LibrarySourceBlock=SimscapeFPGAHIL_lib/Linearized Switch Models/Switch/ic_in
  is : fl_lib/Electrical/Electrical Sensors/Current Sensor
      settings: LibrarySourceBlock=SimscapeFPGAHIL_lib/Linearized Switch Models/Switch/is
  is_out : nesl_utility/PS-Simulink Converter  PhysicalDomain=network_engine_domain  SubClassName=ps_output  LeftPortType=input  RightPortType=output  PseudoPeriodic=off  Frequencies=[]  VectorFormat=1-D array  Unit=A  AffineConversion=off
      settings: LibrarySourceBlock=SimscapeFPGAHIL_lib/Linearized Switch Models/Switch/is_out
  vs : fl_lib/Electrical/Electrical Sensors/Voltage Sensor
      settings: LibrarySourceBlock=SimscapeFPGAHIL_lib/Linearized Switch Models/Switch/vs
  vs_out : nesl_utility/PS-Simulink Converter  PhysicalDomain=network_engine_domain  SubClassName=ps_output  LeftPortType=input  RightPortType=output  PseudoPeriodic=off  Frequencies=[]  VectorFormat=1-D array  Unit=V  AffineConversion=off
      settings: LibrarySourceBlock=SimscapeFPGAHIL_lib/Linearized Switch Models/Switch/vs_out
  + : PMIOPort  Side=Left
  - : PMIOPort  Port=2  Side=Right
  wires:
  Controller/1 -> ic_in/1
  G/1 -> Controller/3
  is_out/1 -> Controller/2
  vs_out/1 -> Controller/1
  connections:
  is_out/LConn1 -- is/RConn1
  vs_out/LConn1 -- vs/RConn1
  ic_in/RConn1 -- ic/RConn1
  is/LConn1 -- +/RConn1 -- vs/LConn1
  ic/RConn2 -- Gs/RConn1 -- -/RConn1 -- vs/RConn2
  is/RConn2 -- Gs/LConn1 -- ic/LConn1

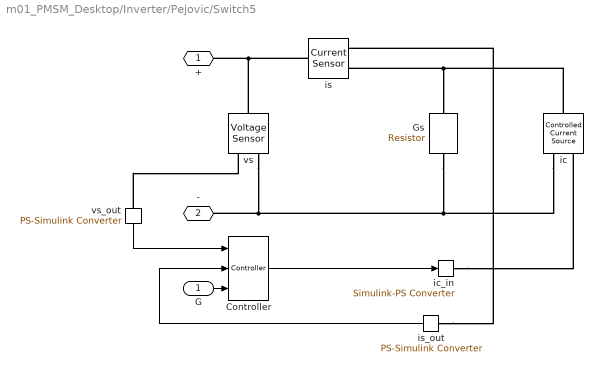
== system m01_PMSM_Desktop/Inverter/Pejovic/Switch5 ==
  G : Inport
  Controller : SimscapeFPGAHIL_lib/Linearized Switch Models/Switch/Controller  threshold=threshold  Gs=Gs  s=timeScaling  avgFactor=avgFactor  isFixedPoint=off
  Gs : fl_lib/Electrical/Electrical Elements/Resistor  R=1/Gs Ohm  i_specify=off  i_priority=None  i=0 A  i_nominal_specify=off  i_nominal_unit=A  i_nominal_value=1  v_specify=off  v_priority=None  v=0 V  v_nominal_specify=off  v_nominal_unit=V  v_nominal_value=1
      settings: LibrarySourceBlock=SimscapeFPGAHIL_lib/Linearized Switch Models/Switch/Gs
  ic : fl_lib/Electrical/Electrical Sources/Controlled Current Source
      settings: LibrarySourceBlock=SimscapeFPGAHIL_lib/Linearized Switch Models/Switch/ic
  ic_in : nesl_utility/Simulink-PS Converter  PhysicalDomain=network_engine_domain  SubClassName=ps_input  LeftPortType=input  RightPortType=output  PseudoPeriodic=off  Frequencies=[]  NoiseDistribution=none  NoiseParameters=[]  Unit=A  AffineConversion=off  FilteringAndDerivatives=provide  SimscapeFilterOrder=1  InputFilterTimeConstant=0.001  UdotUserProvided=0
      settings: LibrarySourceBlock=SimscapeFPGAHIL_lib/Linearized Switch Models/Switch/ic_in
  is : fl_lib/Electrical/Electrical Sensors/Current Sensor
      settings: LibrarySourceBlock=SimscapeFPGAHIL_lib/Linearized Switch Models/Switch/is
  is_out : nesl_utility/PS-Simulink Converter  PhysicalDomain=network_engine_domain  SubClassName=ps_output  LeftPortType=input  RightPortType=output  PseudoPeriodic=off  Frequencies=[]  VectorFormat=1-D array  Unit=A  AffineConversion=off
      settings: LibrarySourceBlock=SimscapeFPGAHIL_lib/Linearized Switch Models/Switch/is_out
  vs : fl_lib/Electrical/Electrical Sensors/Voltage Sensor
      settings: LibrarySourceBlock=SimscapeFPGAHIL_lib/Linearized Switch Models/Switch/vs
  vs_out : nesl_utility/PS-Simulink Converter  PhysicalDomain=network_engine_domain  SubClassName=ps_output  LeftPortType=input  RightPortType=output  PseudoPeriodic=off  Frequencies=[]  VectorFormat=1-D array  Unit=V  AffineConversion=off
      settings: LibrarySourceBlock=SimscapeFPGAHIL_lib/Linearized Switch Models/Switch/vs_out
  + : PMIOPort  Side=Left
  - : PMIOPort  Port=2  Side=Right
  wires:
  vs_out/1 -> Controller/1
  is_out/1 -> Controller/2
  G/1 -> Controller/3
  Controller/1 -> ic_in/1
  connections:
  ic/LConn1 -- Gs/LConn1 -- is/RConn2
  vs/RConn2 -- -/RConn1 -- Gs/RConn1 -- ic/RConn2
  vs/LConn1 -- +/RConn1 -- is/LConn1
  ic_in/RConn1 -- ic/RConn1
  vs_out/LConn1 -- vs/RConn1
  is_out/LConn1 -- is/RConn1

== system m01_PMSM_Desktop/Inverter/Pejovic/Switch6 ==
  G : Inport
  Controller : SimscapeFPGAHIL_lib/Linearized Switch Models/Switch/Controller  threshold=threshold  Gs=Gs  s=timeScaling  avgFactor=avgFactor  isFixedPoint=off
  Gs : fl_lib/Electrical/Electrical Elements/Resistor  R=1/Gs Ohm  i_specify=off  i_priority=None  i=0 A  i_nominal_specify=off  i_nominal_unit=A  i_nominal_value=1  v_specify=off  v_priority=None  v=0 V  v_nominal_specify=off  v_nominal_unit=V  v_nominal_value=1
      settings: LibrarySourceBlock=SimscapeFPGAHIL_lib/Linearized Switch Models/Switch/Gs
  ic : fl_lib/Electrical/Electrical Sources/Controlled Current Source
      settings: LibrarySourceBlock=SimscapeFPGAHIL_lib/Linearized Switch Models/Switch/ic
  ic_in : nesl_utility/Simulink-PS Converter  PhysicalDomain=network_engine_domain  SubClassName=ps_input  LeftPortType=input  RightPortType=output  PseudoPeriodic=off  Frequencies=[]  NoiseDistribution=none  NoiseParameters=[]  Unit=A  AffineConversion=off  FilteringAndDerivatives=provide  SimscapeFilterOrder=1  InputFilterTimeConstant=0.001  UdotUserProvided=0
      settings: LibrarySourceBlock=SimscapeFPGAHIL_lib/Linearized Switch Models/Switch/ic_in
  is : fl_lib/Electrical/Electrical Sensors/Current Sensor
      settings: LibrarySourceBlock=SimscapeFPGAHIL_lib/Linearized Switch Models/Switch/is
  is_out : nesl_utility/PS-Simulink Converter  PhysicalDomain=network_engine_domain  SubClassName=ps_output  LeftPortType=input  RightPortType=output  PseudoPeriodic=off  Frequencies=[]  VectorFormat=1-D array  Unit=A  AffineConversion=off
      settings: LibrarySourceBlock=SimscapeFPGAHIL_lib/Linearized Switch Models/Switch/is_out
  vs : fl_lib/Electrical/Electrical Sensors/Voltage Sensor
      settings: LibrarySourceBlock=SimscapeFPGAHIL_lib/Linearized Switch Models/Switch/vs
  vs_out : nesl_utility/PS-Simulink Converter  PhysicalDomain=network_engine_domain  SubClassName=ps_output  LeftPortType=input  RightPortType=output  PseudoPeriodic=off  Frequencies=[]  VectorFormat=1-D array  Unit=V  AffineConversion=off
      settings: LibrarySourceBlock=SimscapeFPGAHIL_lib/Linearized Switch Models/Switch/vs_out
  + : PMIOPort  Side=Left
  - : PMIOPort  Port=2  Side=Right
  wires:
  Controller/1 -> ic_in/1
  G/1 -> Controller/3
  is_out/1 -> Controller/2
  vs_out/1 -> Controller/1
  connections:
  is_out/LConn1 -- is/RConn1
  vs_out/LConn1 -- vs/RConn1
  ic_in/RConn1 -- ic/RConn1
  is/LConn1 -- +/RConn1 -- vs/LConn1
  ic/RConn2 -- Gs/RConn1 -- -/RConn1 -- vs/RConn2
  is/RConn2 -- Gs/LConn1 -- ic/LConn1

== system m01_PMSM_Desktop/Inverter/Pejovic w//SCA/Switch1 ==
  G : Inport
  Controller : SimscapeFPGAHIL_lib/Linearized Switch Models/Switch/Controller  threshold=threshold  Gs=Gs  s=timeScaling  avgFactor=avgFactor  isFixedPoint=off
  Gs : fl_lib/Electrical/Electrical Elements/Resistor  R=1/Gs Ohm  i_specify=off  i_priority=None  i=0 A  i_nominal_specify=off  i_nominal_unit=A  i_nominal_value=1  v_specify=off  v_priority=None  v=0 V  v_nominal_specify=off  v_nominal_unit=V  v_nominal_value=1
      settings: LibrarySourceBlock=SimscapeFPGAHIL_lib/Linearized Switch Models/Switch/Gs
  ic : fl_lib/Electrical/Electrical Sources/Controlled Current Source
      settings: LibrarySourceBlock=SimscapeFPGAHIL_lib/Linearized Switch Models/Switch/ic
  ic_in : nesl_utility/Simulink-PS Converter  PhysicalDomain=network_engine_domain  SubClassName=ps_input  LeftPortType=input  RightPortType=output  PseudoPeriodic=off  Frequencies=[]  NoiseDistribution=none  NoiseParameters=[]  Unit=A  AffineConversion=off  FilteringAndDerivatives=provide  SimscapeFilterOrder=1  InputFilterTimeConstant=0.001  UdotUserProvided=0
      settings: LibrarySourceBlock=SimscapeFPGAHIL_lib/Linearized Switch Models/Switch/ic_in
  is : fl_lib/Electrical/Electrical Sensors/Current Sensor
      settings: LibrarySourceBlock=SimscapeFPGAHIL_lib/Linearized Switch Models/Switch/is
  is_out : nesl_utility/PS-Simulink Converter  PhysicalDomain=network_engine_domain  SubClassName=ps_output  LeftPortType=input  RightPortType=output  PseudoPeriodic=off  Frequencies=[]  VectorFormat=1-D array  Unit=A  AffineConversion=off
      settings: LibrarySourceBlock=SimscapeFPGAHIL_lib/Linearized Switch Models/Switch/is_out
  vs : fl_lib/Electrical/Electrical Sensors/Voltage Sensor
      settings: LibrarySourceBlock=SimscapeFPGAHIL_lib/Linearized Switch Models/Switch/vs
  vs_out : nesl_utility/PS-Simulink Converter  PhysicalDomain=network_engine_domain  SubClassName=ps_output  LeftPortType=input  RightPortType=output  PseudoPeriodic=off  Frequencies=[]  VectorFormat=1-D array  Unit=V  AffineConversion=off
      settings: LibrarySourceBlock=SimscapeFPGAHIL_lib/Linearized Switch Models/Switch/vs_out
  + : PMIOPort  Side=Left
  - : PMIOPort  Port=2  Side=Right
  wires:
  vs_out/1 -> Controller/1
  is_out/1 -> Controller/2
  G/1 -> Controller/3
  Controller/1 -> ic_in/1
  connections:
  ic/LConn1 -- Gs/LConn1 -- is/RConn2
  vs/RConn2 -- -/RConn1 -- Gs/RConn1 -- ic/RConn2
  vs/LConn1 -- +/RConn1 -- is/LConn1
  ic_in/RConn1 -- ic/RConn1
  vs_out/LConn1 -- vs/RConn1
  is_out/LConn1 -- is/RConn1

== system m01_PMSM_Desktop/Inverter/Pejovic w//SCA/Switch2 ==
  G : Inport
  Controller : SimscapeFPGAHIL_lib/Linearized Switch Models/Switch/Controller  threshold=threshold  Gs=Gs  s=timeScaling  avgFactor=avgFactor  isFixedPoint=off
  Gs : fl_lib/Electrical/Electrical Elements/Resistor  R=1/Gs Ohm  i_specify=off  i_priority=None  i=0 A  i_nominal_specify=off  i_nominal_unit=A  i_nominal_value=1  v_specify=off  v_priority=None  v=0 V  v_nominal_specify=off  v_nominal_unit=V  v_nominal_value=1
      settings: LibrarySourceBlock=SimscapeFPGAHIL_lib/Linearized Switch Models/Switch/Gs
  ic : fl_lib/Electrical/Electrical Sources/Controlled Current Source
      settings: LibrarySourceBlock=SimscapeFPGAHIL_lib/Linearized Switch Models/Switch/ic
  ic_in : nesl_utility/Simulink-PS Converter  PhysicalDomain=network_engine_domain  SubClassName=ps_input  LeftPortType=input  RightPortType=output  PseudoPeriodic=off  Frequencies=[]  NoiseDistribution=none  NoiseParameters=[]  Unit=A  AffineConversion=off  FilteringAndDerivatives=provide  SimscapeFilterOrder=1  InputFilterTimeConstant=0.001  UdotUserProvided=0
      settings: LibrarySourceBlock=SimscapeFPGAHIL_lib/Linearized Switch Models/Switch/ic_in
  is : fl_lib/Electrical/Electrical Sensors/Current Sensor
      settings: LibrarySourceBlock=SimscapeFPGAHIL_lib/Linearized Switch Models/Switch/is
  is_out : nesl_utility/PS-Simulink Converter  PhysicalDomain=network_engine_domain  SubClassName=ps_output  LeftPortType=input  RightPortType=output  PseudoPeriodic=off  Frequencies=[]  VectorFormat=1-D array  Unit=A  AffineConversion=off
      settings: LibrarySourceBlock=SimscapeFPGAHIL_lib/Linearized Switch Models/Switch/is_out
  vs : fl_lib/Electrical/Electrical Sensors/Voltage Sensor
      settings: LibrarySourceBlock=SimscapeFPGAHIL_lib/Linearized Switch Models/Switch/vs
  vs_out : nesl_utility/PS-Simulink Converter  PhysicalDomain=network_engine_domain  SubClassName=ps_output  LeftPortType=input  RightPortType=output  PseudoPeriodic=off  Frequencies=[]  VectorFormat=1-D array  Unit=V  AffineConversion=off
      settings: LibrarySourceBlock=SimscapeFPGAHIL_lib/Linearized Switch Models/Switch/vs_out
  + : PMIOPort  Side=Left
  - : PMIOPort  Port=2  Side=Right
  wires:
  Controller/1 -> ic_in/1
  G/1 -> Controller/3
  is_out/1 -> Controller/2
  vs_out/1 -> Controller/1
  connections:
  is_out/LConn1 -- is/RConn1
  vs_out/LConn1 -- vs/RConn1
  ic_in/RConn1 -- ic/RConn1
  is/LConn1 -- +/RConn1 -- vs/LConn1
  ic/RConn2 -- Gs/RConn1 -- -/RConn1 -- vs/RConn2
  is/RConn2 -- Gs/LConn1 -- ic/LConn1

== system m01_PMSM_Desktop/Inverter/Pejovic w//SCA/Switch3 ==
  G : Inport
  Controller : SimscapeFPGAHIL_lib/Linearized Switch Models/Switch/Controller  threshold=threshold  Gs=Gs  s=timeScaling  avgFactor=avgFactor  isFixedPoint=off
  Gs : fl_lib/Electrical/Electrical Elements/Resistor  R=1/Gs Ohm  i_specify=off  i_priority=None  i=0 A  i_nominal_specify=off  i_nominal_unit=A  i_nominal_value=1  v_specify=off  v_priority=None  v=0 V  v_nominal_specify=off  v_nominal_unit=V  v_nominal_value=1
      settings: LibrarySourceBlock=SimscapeFPGAHIL_lib/Linearized Switch Models/Switch/Gs
  ic : fl_lib/Electrical/Electrical Sources/Controlled Current Source
      settings: LibrarySourceBlock=SimscapeFPGAHIL_lib/Linearized Switch Models/Switch/ic
  ic_in : nesl_utility/Simulink-PS Converter  PhysicalDomain=network_engine_domain  SubClassName=ps_input  LeftPortType=input  RightPortType=output  PseudoPeriodic=off  Frequencies=[]  NoiseDistribution=none  NoiseParameters=[]  Unit=A  AffineConversion=off  FilteringAndDerivatives=provide  SimscapeFilterOrder=1  InputFilterTimeConstant=0.001  UdotUserProvided=0
      settings: LibrarySourceBlock=SimscapeFPGAHIL_lib/Linearized Switch Models/Switch/ic_in
  is : fl_lib/Electrical/Electrical Sensors/Current Sensor
      settings: LibrarySourceBlock=SimscapeFPGAHIL_lib/Linearized Switch Models/Switch/is
  is_out : nesl_utility/PS-Simulink Converter  PhysicalDomain=network_engine_domain  SubClassName=ps_output  LeftPortType=input  RightPortType=output  PseudoPeriodic=off  Frequencies=[]  VectorFormat=1-D array  Unit=A  AffineConversion=off
      settings: LibrarySourceBlock=SimscapeFPGAHIL_lib/Linearized Switch Models/Switch/is_out
  vs : fl_lib/Electrical/Electrical Sensors/Voltage Sensor
      settings: LibrarySourceBlock=SimscapeFPGAHIL_lib/Linearized Switch Models/Switch/vs
  vs_out : nesl_utility/PS-Simulink Converter  PhysicalDomain=network_engine_domain  SubClassName=ps_output  LeftPortType=input  RightPortType=output  PseudoPeriodic=off  Frequencies=[]  VectorFormat=1-D array  Unit=V  AffineConversion=off
      settings: LibrarySourceBlock=SimscapeFPGAHIL_lib/Linearized Switch Models/Switch/vs_out
  + : PMIOPort  Side=Left
  - : PMIOPort  Port=2  Side=Right
  wires:
  vs_out/1 -> Controller/1
  is_out/1 -> Controller/2
  G/1 -> Controller/3
  Controller/1 -> ic_in/1
  connections:
  ic/LConn1 -- Gs/LConn1 -- is/RConn2
  vs/RConn2 -- -/RConn1 -- Gs/RConn1 -- ic/RConn2
  vs/LConn1 -- +/RConn1 -- is/LConn1
  ic_in/RConn1 -- ic/RConn1
  vs_out/LConn1 -- vs/RConn1
  is_out/LConn1 -- is/RConn1
